simulink model "feedback_lin_RLS_Template_2023"  (R2023b)
settings: Solver=ode1  StartTime=0.0  StopTime=inf  FixedStep=0.002  RelTol=1e-3  EnableMultiTasking=on
PostLoadFcn:
  | qc_set_target_type(getConfigSet(bdroot, 'QUARC Default Target Configuration'));
values from neighbouring files (symbols this model uses):
  A_ob = A - L*C    [main_feedback_lin.m]
  B_ob = [ B - L*D, L]    [main_feedback_lin.m]
  C_ob = eye(n)    [main_feedback_lin.m]
  D_ob = zeros(n, q+p)    [main_feedback_lin.m]
  k_mag_mod = 3.4405e-05    [main_feedback_lin.m]
  Lc_mod = 0.3708    [main_feedback_lin.m]
  Rtot_mod = 7.7585    [main_feedback_lin.m]
undefined symbols (not defined in the file or in its folder): HIL, k_aero, k_mag, Kb, Lc, m, offset_corrente_volt, offset_posizione_volt, Rtot, x1_eq0, x2_eq0, y0
libraries: quarc_library x4, slpidlib x1
settings Model: SimulationMode=external  ExtModeTrigDuration=5000  Creator=CFulford  LastModifiedBy=lollo
settings SolverCC: AlgebraicLoopSolver=TrustRegion  PositivePriorityOrder=on
settings DataIOCC: LimitDataPoints=on  SaveFormat=Array  SignalLoggingSaveFormat=ModelDataLogs  ReturnWorkspaceOutputs=off
settings OptimizationCC: ExpressionDepthLimit=2147483647  InitFltsAndDblsToZero=on  LifeSpan=inf
settings DebuggingCC: SaveWithParameterizedLinksMsg=none  UnderspecifiedInitializationDetection=Classic  MergeDetectMultiDrivingBlocksExec=none  SolverPrmCheckMsg=warning  MultiTaskDSMMsg=warning  MultiTaskCondExecSysMsg=none  FcnCallInpInsideContextMsg=warning  UnconnectedInputMsg=warning  UnconnectedOutputMsg=warning  UnconnectedLineMsg=warning  StateNameClashWarn=warning  SFUnexpectedBacktrackingDiag=warning  SFNoUnconditionalDefaultTransitionDiag=warning  SFExecutionAtInitializationDiag=none  ArithmeticOperatorsInVariantConditions=warning
settings HardwareCC: ProdBitPerPointer=32  ProdBitPerSizeT=32  ProdBitPerPtrDiffT=32  ProdLargestAtomicFloat=None  ProdIntDivRoundTo=Undefined  ProdEndianess=Unspecified  ProdWordSize=32  ProdHWDeviceType=32-bit Generic
settings ModelReferenceCC: EnableRefExpFcnMdlSchedulingChecks=on  PropagateSignalLabelsOutOfModel=off
settings SFSimCC: SimUseLocalCustomCode=off  CustomCodeUndefinedFunction=UseInterfaceOnly
settings RTWCC: Description=QUARC Win64 Target  SystemTargetFile=quarc_win64.tlc  TemplateMakefile=quarc_default_tmf  RTWUseLocalCustomCode=off
settings CodeAppCC: StateflowObjectComments=on
settings STFCustomTargetCC: TargetPreCompLibLocation=C:\PROGRA~3\QUARC\lib\2019b\win64\release  TargetLangStandard=C89/C90 (ANSI)  ConcurrentExecutionCompliant=on  CombineOutputUpdateFcns=on  CPPClassGenCompliant=on  SystemTargetFile=quarc_win64.tlc
settings GRTTargetCC: TargetPreCompLibLocation=C:\PROGRA~3\QUARC\lib\2019b\win64\release  TargetLangStandard=C89/C90 (ANSI)  ParMdlRefBuildCompliant=off  CompOptLevelCompliant=off  MatFileLogging=off  UseToolchainInfoCompliant=off  ExtMode=on  ExtModeMexFile=quarc_comm
settings ConfigComp: CovMetricSettings=dw  CovSaveCumulativeToWorkspaceVar=on  CovSaveSingleToWorkspaceVar=on  CovExternalEMLEnable=off  CovSFcnEnable=off

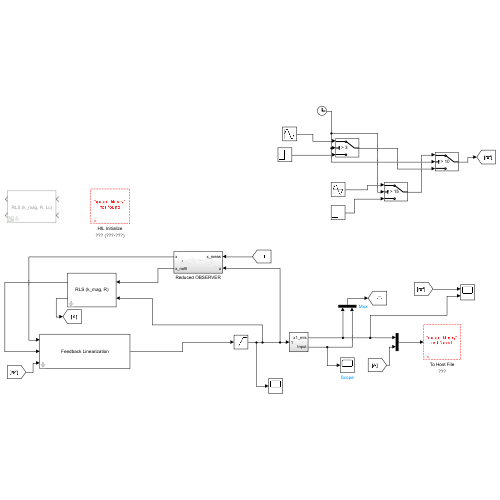
[thumbnail: Simulink's stored preview of the top-level diagram]
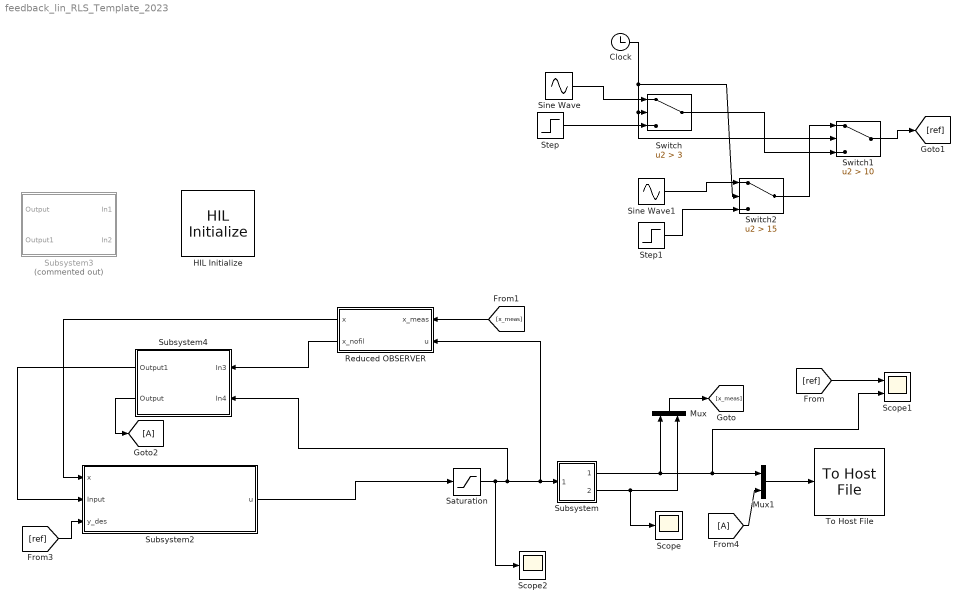
== system feedback_lin_RLS_Template_2023 ==
  Clock : Clock
  From4 : From
  Goto2 : Goto
  HIL Initialize : quarc_library/Data Acquisition/Generic/Configuration/HIL Initialize  Priority=-99  object_name=HIL-1  board_type=q2_usb  board_number=0  board_options=d0=digital;d1=digital;led=auto;update_rate=normal;decimation=1  exclusive=off  active=off  hardware_clocks=[0]  clock_modes=[]  initial_clock_frequencies=[]  set_clock_params_at_start=off  set_clock_params_at_switch_in=off  set_clock_frequencies_at_start=off  set_clock_frequencies_at_switch_in=off  analog_input_channels=[0:1]  analog_input_configurations=[]  analog_input_maximums=10  analog_input_minimums=-10  set_analog_input_params_at_start=on  set_analog_input_params_at_switch_in=off  analog_output_channels=[0:1]  analog_output_maximums=10  analog_output_minimums=-10  initial_analog_outputs=[0]  final_analog_outputs=[0]  watchdog_analog_outputs=0  set_analog_output_params_at_start=on  set_analog_output_params_at_switch_in=off  set_analog_outputs_at_start=on  set_analog_outputs_at_switch_in=off  set_analog_outputs_at_terminate=on  set_analog_outputs_at_switch_out=off  set_analog_outputs_on_watchdog=off  digital_input_channels=[]  digital_output_channels=[]  digital_output_configuration=[]  initial_digital_outputs=[1]  final_digital_outputs=[1]  watchdog_digital_outputs=[1]  set_digital_output_params_at_start=off  set_digital_output_params_at_switch_in=off  set_digital_outputs_at_start=on  set_digital_outputs_at_switch_in=off  set_digital_outputs_at_terminate=on  set_digital_outputs_at_switch_out=off  set_digital_outputs_on_watchdog=off  encoder_channels=[0:1]  quadrature=[4]  encoder_filter_frequency=[]  initial_encoder_counts=[0]  set_encoder_params_at_start=on  set_encoder_params_at_switch_in=off  set_encoder_counts_at_start=on  set_encoder_counts_at_switch_in=off  pwm_channels=[]  pwm_modes=[0]  pwm_frequency=1/0.020  pwm_configuration=[]  pwm_alignment=[]  pwm_polarity=[]  pwm_leading_deadband=[]  pwm_trailing_deadband=[]  initial_pwm_outputs=[0]  final_pwm_outputs=[0]  watchdog_pwm_outputs=[0]  set_pwm_params_at_start=on  set_pwm_params_at_switch_in=off  set_pwm_outputs_at_start=on  set_pwm_outputs_at_switch_in=off  set_pwm_outputs_at_terminate=on  set_pwm_outputs_at_switch_out=off  set_pwm_outputs_on_watchdog=off  other_output_channels=[]  initial_other_outputs=[]  final_other_outputs=[]  watchdog_other_outputs=[]  set_other_outputs_at_start=off  set_other_outputs_at_switch_in=off  set_other_outputs_at_terminate=off  set_other_outputs_at_switch_out=off  set_other_outputs_on_watchdog=off
  Mux : Mux  Inputs=2
  Mux1 : Mux  Inputs=2
  Reduced OBSERVER : Subsystem
  Saturation : Saturate  UpperLimit=23  LowerLimit=0
  Scope : Scope
  Scope1 : Scope  NumInputPorts=2
  Scope2 : Scope
  Sine Wave : Sin  Amplitude=0.0008  Bias=0.004  Frequency=10  SampleTime=0
  Sine Wave1 : Sin  Amplitude=0.0005  Bias=0.004  Frequency=10  SampleTime=0
  Step : Step  Time=2  After=0.004  SampleTime=0
  Step1 : Step  Time=2  After=0.003  SampleTime=0
  Subsystem : Subsystem
  Subsystem2 : Subsystem  mask{tau=0.003, p1=-100, p2=-60, p3=-70}
      mask DialogControl DescGroupVar Prompt: Feedback Linearization
      mask DialogControl DescTextVar Prompt: Tau corrisponde al tempo caratteristico del filtro per il calcolo delle derivate. k1, k2, k3 sono i poli della feedback linearization dei rispettivi stati
      mask Display: disp('Feedback Linearization')
  Subsystem3 : Subsystem  Commented=on
      mask Display: disp('RLS (k_mag, R, Lc)')
  Subsystem4 : Subsystem
      mask Display: disp('RLS (k_mag, R)')
  Switch : Switch  Criteria=u2 > Threshold  Threshold=3  SaturateOnIntegerOverflow=off  InputSameDT=off
  Switch1 : Switch  Criteria=u2 > Threshold  Threshold=10  SaturateOnIntegerOverflow=off  InputSameDT=off
  Switch2 : Switch  Criteria=u2 > Threshold  Threshold=15  SaturateOnIntegerOverflow=off  InputSameDT=off
  To Host File : quarc_library/Sinks/To Host/To Host File  file_name=data_%{date}_%{time}.mat  variable_name=data_%{date}_%{time}  decimation=1  sample_time=-1  file_format=MAT-file v.5  options=No header or footer  append=off  final_file_name=data_23-May-2025_13-05-44.mat  bitrate=2000000
  wires:
  Saturation/1 -> Scope2/1, Subsystem4/2(In4), Reduced OBSERVER/2(u), Subsystem/1(In1)
  Subsystem/2(Input) -> Mux/2, Scope/1
  Mux1/1 -> To Host File/1
  Subsystem2/1(u) -> Saturation/1
  [x_meas] -> Reduced OBSERVER/1(x_meas)
  Reduced OBSERVER/2(x_nofil) -> Subsystem4/1(In3)
  Reduced OBSERVER/1(x) -> Subsystem2/1(x)
  Subsystem4/1(Output1) -> Subsystem2/2(Input)
  Sine Wave/1 -> Switch/1
  Step/1 -> Switch/3
  [ref] -> Subsystem2/3(y_des)
  Subsystem4/2(Output) -> Goto2/1
  From4/1 -> Mux1/2
  Mux/1 -> [x_meas]
  Step1/1 -> Switch2/3
  Sine Wave1/1 -> Switch2/1
  Switch/1 -> Switch1/3
  Switch2/1 -> Switch1/1
  Clock/1 -> Switch1/2, Switch/2, Switch2/2
  Switch1/1 -> [ref]
  [ref] -> Scope1/1
  Subsystem/1(x1_mis) -> Scope1/2, Mux1/1, Mux/1

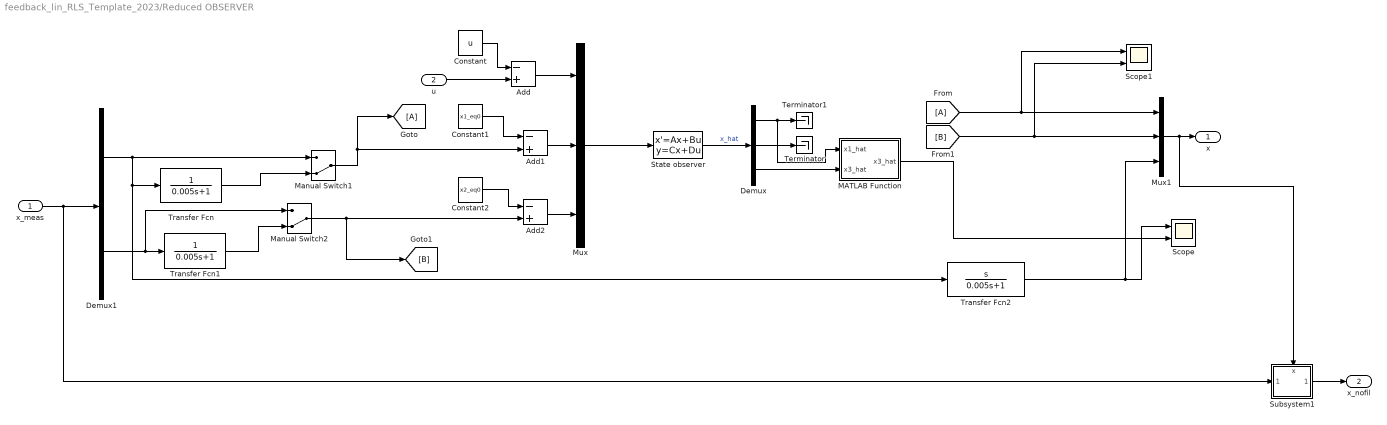
== system feedback_lin_RLS_Template_2023/Reduced OBSERVER ==
  x_meas : Inport
  u : Inport  Port=2
  Add : Sum  Inputs=-+
  Add1 : Sum  Inputs=-+
  Add2 : Sum  Inputs=-+
  Constant : Constant  Value=u
  Constant1 : Constant  Value=x1_eq0
  Constant2 : Constant  Value=x2_eq0
  Demux : Demux  Outputs=3
  Demux1 : Demux  Outputs=2
  From : From
  Goto : Goto
  MATLAB Function : MATLAB Function  TreatAsAtomicUnit=on
  Manual Switch1 : ManualSwitch  CurrentSetting=0
  Manual Switch2 : ManualSwitch  CurrentSetting=0
  Mux : Mux  Inputs=3
  Mux1 : Mux  Inputs=3
  Scope : Scope  NumInputPorts=2
  Scope1 : Scope  NumInputPorts=2
  State observer : StateSpace  A=A_ob  B=B_ob  C=C_ob  D=D_ob  InitialCondition=[0;0;0]
  Subsystem1 : Subsystem
      settings: PortSchema="{\"entries\":[{\"content\":{\"sides\":[{\"content\":{\"connectorIds\":[\"In1\"]},\"type\":\"ConnectorPlacement.EquallySpacedRectSide\",\"uuid\":\"f48180fa-4225-4978-addf-748f5b56b5ff\"},{\"content\":{\"connectorIds\":[\"Out1\"],\"side\":\"RIGHT\"},\"type\":\"ConnectorPlacement.EquallySpacedRectSide\",\"uuid\":\"29b082be-84d5-4b73-aaf8-582ec952e070\"},{\"content\":{\"connectorIds\":[\"In2\"],\"side\":\"TOP\"},\"type\":\"ConnectorPlacement.EquallySpacedRectSide\",\"uuid\":\"6e43ab95-1f09-4bed-ac58-60c8e8d5deec\"}]},\"type\":\"ConnectorPlacement.EquallySpacedConnector\",\"uuid\":\"d6520a9c-dc2f-4cc0-9c8c-cd26f1cfe6f6\"}],\"packageUris\":[\"http://schema.mathworks.com/mf0/Connector/R2020b\"],\"version\":\"1.0\"}"
  Terminator : Terminator
  Terminator1 : Terminator
  Transfer Fcn : TransferFcn  Denominator=[0.005 1]
  Transfer Fcn1 : TransferFcn  Denominator=[0.005 1]
  Transfer Fcn2 : TransferFcn  Numerator=[1 0]  Denominator=[0.005 1]
  x : Outport
  x_nofil : Outport  Port=2
  wires:
  u/1 -> Add/2
  Mux/1 -> State observer/1
  State observer/1 -> Demux/1  "x_hat"
  Demux/1 -> Terminator1/1, MATLAB Function/1(x1_hat)
  Constant/1 -> Add/1
  Constant1/1 -> Add1/1
  Constant2/1 -> Add2/1
  Add/1 -> Mux/1
  Add1/1 -> Mux/2
  Add2/1 -> Mux/3
  Demux/3 -> MATLAB Function/2("x3_hat ")
  Mux1/1 -> Subsystem1/2(x), x/1
  MATLAB Function/1(x3_hat) -> Scope/2
  Demux/2 -> Terminator/1
  x_meas/1 -> Subsystem1/1(x_meas), Demux1/1
  [B] -> Scope1/2, Mux1/2
  From/1 -> Scope1/1, Mux1/1
  Transfer Fcn/1 -> Manual Switch1/2
  Demux1/1 -> Transfer Fcn2/1, Transfer Fcn/1, Manual Switch1/1
  Manual Switch1/1 -> Add1/2, Goto/1
  Transfer Fcn1/1 -> Manual Switch2/2
  Demux1/2 -> Manual Switch2/1, Transfer Fcn1/1
  Manual Switch2/1 -> Add2/2, [B]
  Transfer Fcn2/1 -> Mux1/3, Scope/1
  Subsystem1/1(Out1) -> x_nofil/1

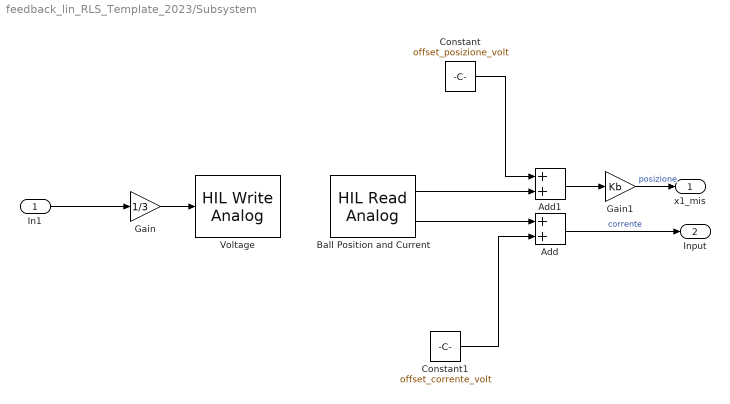
== system feedback_lin_RLS_Template_2023/Subsystem ==
  In1 : Inport
  Add : Sum
  Add1 : Sum
  Ball Position and Current : quarc_library/Data Acquisition/Generic/Immediate I//O/HIL Read Analog  object_name=HIL-1  channels=[0:1]  sample_time=qc_get_step_size  active=on  vector_output=off
  Constant : Constant  Value=offset_posizione_volt
  Constant1 : Constant  Value=offset_corrente_volt
  Gain : Gain  Gain=1/3
  Gain1 : Gain  Gain=Kb
  Voltage : quarc_library/Data Acquisition/Generic/Immediate I//O/HIL Write Analog  object_name=HIL-1  channels=0  sample_time=-1  active=off  vector_input=off
  x1_mis : Outport
  Input : Outport  Port=2
  wires:
  Ball Position and Current/1 -> Add1/2
  In1/1 -> Gain/1
  Ball Position and Current/2 -> Add/1
  Gain/1 -> Voltage/1
  Gain1/1 -> x1_mis/1  "posizione"
  Add1/1 -> Gain1/1
  Add/1 -> Input/1  "corrente"
  Constant1/1 -> Add/2
  Constant/1 -> Add1/1

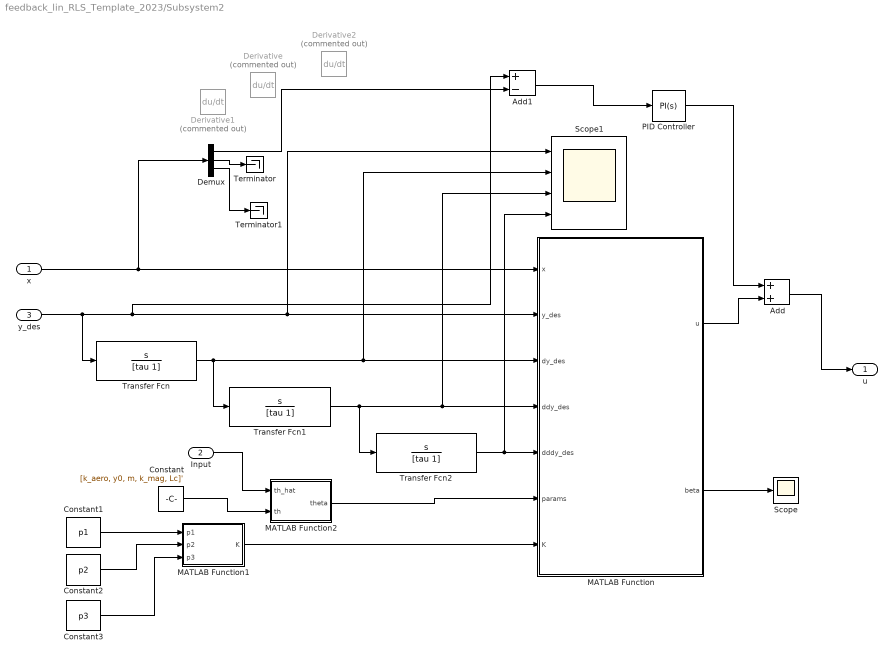
== system feedback_lin_RLS_Template_2023/Subsystem2 ==
  x : Inport
  Input : Inport  Port=2
  y_des : Inport  Port=3
  Add : Sum
  Add1 : Sum  Inputs=+-
  Constant : Constant  Value=[k_aero, y0, m, k_mag, Lc]'
  Constant1 : Constant  Value=p1
  Constant2 : Constant  Value=p2
  Constant3 : Constant  Value=p3
  Demux : Demux  Outputs=3
  Derivative : Derivative  Commented=on
  Derivative1 : Derivative  Commented=on
  Derivative2 : Derivative  Commented=on
  MATLAB Function : MATLAB Function  TreatAsAtomicUnit=on
  MATLAB Function1 : MATLAB Function  TreatAsAtomicUnit=on
  MATLAB Function2 : MATLAB Function  TreatAsAtomicUnit=on
  PID Controller : slpidlib/PID Controller  Controller=PI  Form=Parallel  TimeDomain=Continuous-time  UseExternalTs=off  SampleTime=-1  IntegratorMethod=Forward Euler  FilterMethod=Forward Euler  ControllerParametersSource=internal  P=1e2  I=3e3  UseKiTs=off  D=0  N=100  UseFilter=on  TunerSelectOption=Transfer Function Based (PID Tuner App)  InitialConditionSource=internal  InitialConditionForIntegrator=0  InitialConditionForFilter=0  DifferentiatorICPrevScaledInput=0  ExternalReset=none  TrackingMode=off  Kt=1  LimitOutput=off  SatLimitsSource=internal  UpperSaturationLimit=inf  LowerSaturationLimit=-inf  LinearizeAsGain=on  AntiWindupMode=none  Kb=1  LimitIntegrator=off  UpperIntegratorSaturationLimit=inf  LowerIntegratorSaturationLimit=-inf  POutMin=[]  POutMax=[]  IOutMin=[]  IOutMax=[]  DOutMin=[]  DOutMax=[]  NOutMin=[]  NOutMax=[]  SumOutMin=[]  SumOutMax=[]  SaturationOutMin=[]  SaturationOutMax=[]  PParamMin=[]  PParamMax=[]  IParamMin=[]  IParamMax=[]  DParamMin=[]  DParamMax=[]  NParamMin=[]  NParamMax=[]  KbParamMin=[]  KbParamMax=[]  KtParamMin=[]  KtParamMax=[]  KbOutMin=[]  KbOutMax=[]  KtOutMin=[]  KtOutMax=[]  IntegratorOutMin=[]  IntegratorOutMax=[]  FilterOutMin=[]  FilterOutMax=[]  SumI1OutMin=[]  SumI1OutMax=[]  SumI2OutMin=[]  SumI2OutMax=[]  SumI3OutMin=[]  SumI3OutMax=[]  SumI4OutMin=[]  SumI4OutMax=[]  SumDOutMin=[]  SumDOutMax=[]  DifferentiatorOutMin=[]  DifferentiatorOutMax=[]  FilterDiffOutCoefMin=[]  FilterDiffOutCoefMax=[]  ReciprocalOutMin=[]  ReciprocalOutMax=[]  SumDenOutMin=[]  SumDenOutMax=[]  SumNumOutMin=[]  SumNumOutMax=[]  DivideOutMin=[]  DivideOutMax=[]  UdiffTsProdOutMin=[]  UdiffTsProdOutMax=[]  NTsProdOutMin=[]  NTsProdOutMax=[]  UintegralTsProdOutMin=[]  UintegralTsProdOutMax=[]  UngainTsProdOutMin=[]  UngainTsProdOutMax=[]  ClampingZeroOutDataTypeStr=Inherit: Inherit via back propagation  ClampingZeroOutMin=[]  ClampingZeroOutMax=[]  FilterDenConstantOutDataTypeStr=Inherit: Inherit via back propagation  FilterDenConstantOutMin=[]  FilterDenConstantOutMax=[]  PCopyOutDataTypeStr=Inherit: Inherit via back propagation  PCopyOutMin=[]  PCopyOutMax=[]  NCopyOutDataTypeStr=Inherit: Inherit via back propagation  NCopyOutMin=[]  NCopyOutMax=[]  IntegratorContinuousStateAttributes=''  IntegratorStateMustResolveToSignalObject=off  IntegratorRTWStateStorageClass=Auto  FilterContinuousStateAttributes=''  FilterStateMustResolveToSignalObject=off  FilterRTWStateStorageClass=Auto  ParallelPVariant=InternalParameters  IdealPVariant=Disabled  IVariant=InternalParameters  DVariant=Disabled  IntegratorVariant=Continuous  SatVariant=Disabled  AWVariant=Passthrough  PCopyVariant=Disabled  TRVariant=Disabled  FdbkBlocksVariant=Forward  IdealPFdbkVariant=Disabled  SatFdbkVariant=Disabled  DerivativeFilterVariant=Disabled  NVariant=Disabled  NCopyVariant=Disabled_SignalSpec  FilterICVariant=Disabled  IntegratorICVariant=InternalICs  ExternalResetVariant=Disabled  TRSumVariant=Passthrough  SumFdbkVariant=Disabled  SumVariant=Sum_PI  TsampFilterVariant=InternalTs  TsampNgainVariant=Passthrough  TsampIntegralVariant=Disabled_SignalSpec  ExternalSaturationOutDataTypeStr=Inherit: Same as second input
  Scope : Scope
  Scope1 : Scope  NumInputPorts=4
  Terminator : Terminator
  Terminator1 : Terminator
  Transfer Fcn : TransferFcn  Numerator=[1 0]  Denominator=[tau 1]
  Transfer Fcn1 : TransferFcn  Numerator=[1 0]  Denominator=[tau 1]
  Transfer Fcn2 : TransferFcn  Numerator=[1 0]  Denominator=[tau 1]
  u : Outport
  wires:
  y_des/1 -> Transfer Fcn/1, Add1/1, MATLAB Function/2(y_des), Scope1/1
  x/1 -> Demux/1, MATLAB Function/1(x)
  MATLAB Function/1(u) -> Add/2
  Transfer Fcn/1 -> MATLAB Function/3(dy_des), Scope1/2, Transfer Fcn1/1
  MATLAB Function2/1(theta) -> MATLAB Function/6(params)
  Transfer Fcn1/1 -> Transfer Fcn2/1, Scope1/3, MATLAB Function/4(ddy_des)
  MATLAB Function/2(beta) -> Scope/1
  Transfer Fcn2/1 -> Scope1/4, MATLAB Function/5(dddy_des)
  MATLAB Function1/1(K) -> MATLAB Function/7(K)
  Constant3/1 -> MATLAB Function1/3(p3)
  Constant2/1 -> MATLAB Function1/2(p2)
  Constant1/1 -> MATLAB Function1/1(p1)
  Input/1 -> MATLAB Function2/1(th_hat)
  Constant/1 -> MATLAB Function2/2(th)
  Add/1 -> u/1
  PID Controller/1 -> Add/1
  Demux/1 -> Add1/2
  Demux/2 -> Terminator/1
  Demux/3 -> Terminator1/1
  Add1/1 -> PID Controller/1

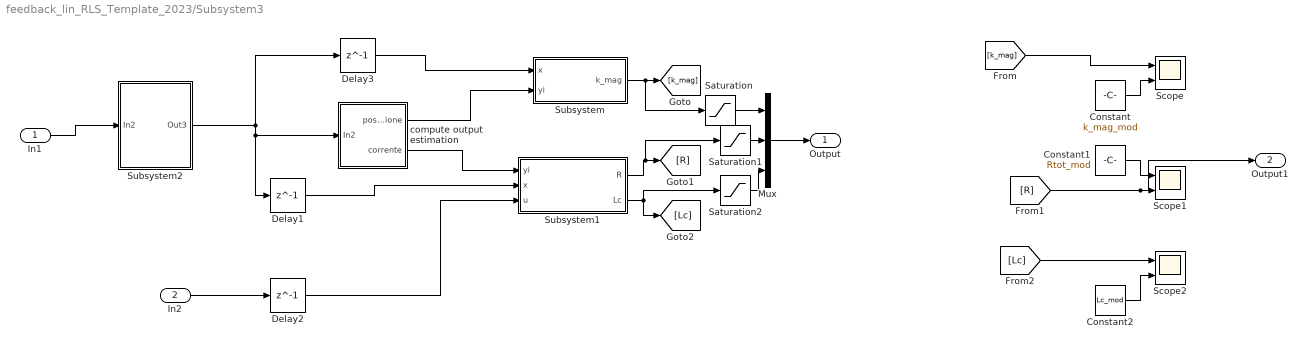
== system feedback_lin_RLS_Template_2023/Subsystem3 ==
  In1 : Inport
  In2 : Inport  Port=2
  Constant : Constant  Value=k_mag_mod
  Constant1 : Constant  Value=Rtot_mod
  Constant2 : Constant  Value=Lc_mod
  Delay1 : Delay  DelayLength=1  InitialCondition=0
  Delay2 : Delay  DelayLength=1  InitialCondition=0
  Delay3 : Delay  DelayLength=1  InitialCondition=[0, 0, 0]'
  Mux : Mux  Inputs=3
  Saturation : Saturate  UpperLimit=1e-4  LowerLimit=1e-6
  Saturation1 : Saturate  UpperLimit=13  LowerLimit=0
  Saturation2 : Saturate  UpperLimit=2  LowerLimit=0
  Scope : Scope  NumInputPorts=2
  Scope1 : Scope  NumInputPorts=2
  Scope2 : Scope  NumInputPorts=2
  Subsystem : Subsystem  mask{th0=k_mag, S0=eye(1)/100, mu=0.98}
      mask prompts: th0 "Theta init"; mu "Forgetting factor"
      mask Display: disp('RLS (k_mag)')
  Subsystem1 : Subsystem  mask{th0=[Rtot; Lc], S0=eye(2)/10, mu=0.99}
      mask prompts: th0 "Theta init"; mu "Forgetting Factor"
      mask Display: disp('RLS (R, Lc)')
  Subsystem2 : Subsystem
  compute output estimation : Subsystem
  Output : Outport
  Output1 : Outport  Port=2
  wires:
  In2/1 -> Delay2/1
  Delay2/1 -> Subsystem1/3(u)
  Delay3/1 -> Subsystem/1(x)
  compute output estimation/1(posizione) -> Subsystem/2(yi)
  compute output estimation/2(corrente) -> Subsystem1/1(yi)
  Delay1/1 -> Subsystem1/2(x)
  Constant/1 -> Scope/2
  Constant1/1 -> Scope1/1
  Constant2/1 -> Scope2/2
  Subsystem/1(k_mag) -> Saturation/1, [k_mag]
  Subsystem1/1(R) -> Saturation1/1, [R]
  Subsystem1/2(Lc) -> [Lc], Saturation2/1
  [k_mag] -> Scope/1
  [R] -> Output1/1, Scope1/2
  [Lc] -> Scope2/1
  Mux/1 -> Output/1
  Subsystem2/1(Out3) -> Delay1/1, compute output estimation/1(In2), Delay3/1
  In1/1 -> Subsystem2/1(In2)
  Saturation/1 -> Mux/1
  Saturation1/1 -> Mux/2
  Saturation2/1 -> Mux/3

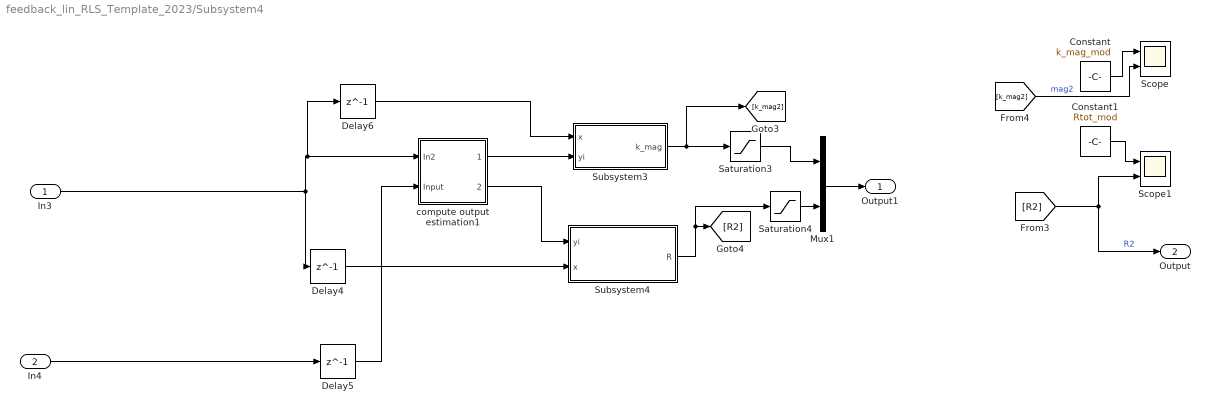
== system feedback_lin_RLS_Template_2023/Subsystem4 ==
  In3 : Inport
  In4 : Inport  Port=2
  Constant : Constant  Value=k_mag_mod
  Constant1 : Constant  Value=Rtot_mod
  Delay4 : Delay  DelayLength=1  InitialCondition=0
  Delay5 : Delay  DelayLength=1  InitialCondition=0
  Delay6 : Delay  DelayLength=1  InitialCondition=[0, 0, 0]'
  Mux1 : Mux  Inputs=2
  Saturation3 : Saturate  UpperLimit=1e-4  LowerLimit=1e-6
  Saturation4 : Saturate  UpperLimit=20  LowerLimit=0
  Scope : Scope  NumInputPorts=2
  Scope1 : Scope  NumInputPorts=2
  Subsystem3 : Subsystem  mask{th0=k_mag, S0=eye(1)/100, mu=0.98}
      mask prompts: th0 "Theta init"; mu "Forgetting factor"
      mask Display: disp('RLS (k_mag)')
  Subsystem4 : Subsystem  mask{th0=Rtot, S0=eye(1)/10, mu=0.99}
      mask prompts: th0 "Theta init"; mu "Forgetting Factor"
      mask Display: disp('RLS (R, Lc)')
  compute output estimation1 : Subsystem
  Output1 : Outport
  Output : Outport  Port=2
  wires:
  Constant/1 -> Scope/1
  Constant1/1 -> Scope1/1
  In3/1 -> Delay4/1, Delay6/1, compute output estimation1/1(In2)
  Saturation4/1 -> Mux1/2
  Subsystem4/1(R) -> Saturation4/1, [R2]
  Delay4/1 -> Subsystem4/2(x)
  Mux1/1 -> Output1/1
  compute output estimation1/2(corrente) -> Subsystem4/1(yi)
  In4/1 -> Delay5/1
  Delay5/1 -> compute output estimation1/2(Input)
  compute output estimation1/1(posizione) -> Subsystem3/2(yi)
  Subsystem3/1(k_mag) -> [k_mag2], Saturation3/1
  Saturation3/1 -> Mux1/1
  Delay6/1 -> Subsystem3/1(x)
  [R2] -> Scope1/2, Output/1  "R2"
  [k_mag2] -> Scope/2  "mag2"

== system feedback_lin_RLS_Template_2023/Reduced OBSERVER/Subsystem1 ==
  x_meas : Inport
  x : Inport  Port=2
  Demux : Demux  Outputs=2
  Demux1 : Demux  Outputs=3
  Mux : Mux  Inputs=3
  Terminator1 : Terminator
  Terminator2 : Terminator
  Out1 : Outport
  wires:
  x/1 -> Demux1/1
  x_meas/1 -> Demux/1
  Demux1/1 -> Terminator1/1
  Demux1/2 -> Terminator2/1
  Mux/1 -> Out1/1
  Demux/1 -> Mux/1
  Demux/2 -> Mux/2
  Demux1/3 -> Mux/3

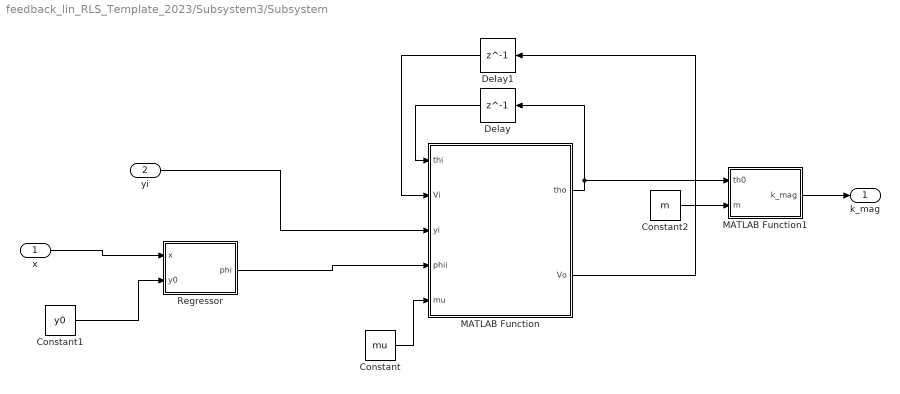
== system feedback_lin_RLS_Template_2023/Subsystem3/Subsystem ==
  x : Inport
  yi : Inport  Port=2
  Constant : Constant  Value=mu
  Constant1 : Constant  Value=y0
  Constant2 : Constant  Value=m
  Delay : Delay  DelayLength=1  InitialCondition=th0*0.002^2/m
  Delay1 : Delay  DelayLength=1  InitialCondition=inv(S0)
  MATLAB Function : MATLAB Function  TreatAsAtomicUnit=on
  MATLAB Function1 : MATLAB Function  TreatAsAtomicUnit=on
  Regressor : MATLAB Function  TreatAsAtomicUnit=on
  k_mag : Outport
  wires:
  yi/1 -> MATLAB Function/3(yi)
  Constant/1 -> MATLAB Function/5(mu)
  Delay/1 -> MATLAB Function/1(thi)
  Delay1/1 -> MATLAB Function/2(Vi)
  MATLAB Function/1(tho) -> MATLAB Function1/1(th0), Delay/1
  Regressor/1(phi) -> MATLAB Function/4(phii)
  MATLAB Function/2(Vo) -> Delay1/1
  x/1 -> Regressor/1(x)
  Constant1/1 -> Regressor/2(y0)
  MATLAB Function1/1(k_mag) -> k_mag/1
  Constant2/1 -> MATLAB Function1/2(m)

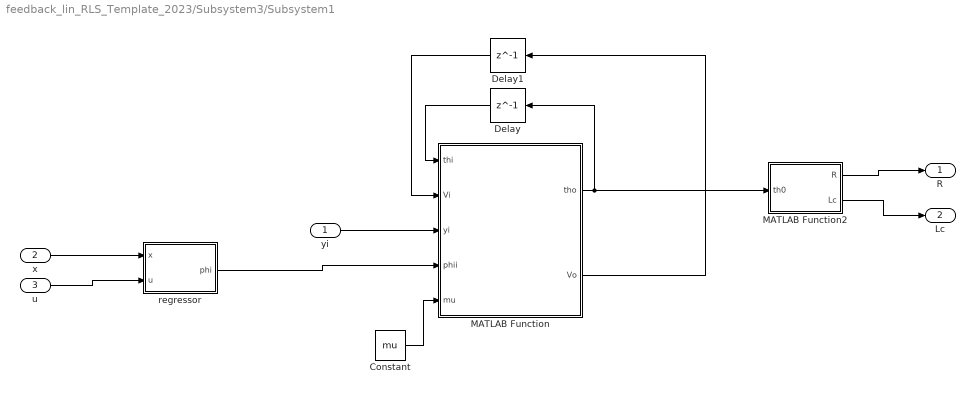
== system feedback_lin_RLS_Template_2023/Subsystem3/Subsystem1 ==
  yi : Inport
  x : Inport  Port=2
  u : Inport  Port=3
  Constant : Constant  Value=mu
  Delay : Delay  DelayLength=1  InitialCondition=[th0(1)*0.002/th0(2); 0.002/th0(2)]
  Delay1 : Delay  DelayLength=1  InitialCondition=inv(S0)
  MATLAB Function : MATLAB Function  TreatAsAtomicUnit=on
  MATLAB Function2 : MATLAB Function  TreatAsAtomicUnit=on
  regressor : MATLAB Function  TreatAsAtomicUnit=on
  R : Outport
  Lc : Outport  Port=2
  wires:
  yi/1 -> MATLAB Function/3(yi)
  Constant/1 -> MATLAB Function/5(mu)
  Delay/1 -> MATLAB Function/1(thi)
  Delay1/1 -> MATLAB Function/2(Vi)
  MATLAB Function/1(tho) -> MATLAB Function2/1(th0), Delay/1
  regressor/1(phi) -> MATLAB Function/4(phii)
  MATLAB Function/2(Vo) -> Delay1/1
  x/1 -> regressor/1(x)
  u/1 -> regressor/2(u)
  MATLAB Function2/1(R) -> R/1
  MATLAB Function2/2(Lc) -> Lc/1

== system feedback_lin_RLS_Template_2023/Subsystem3/Subsystem2 ==
  In2 : Inport
  Demux : Demux  Outputs=3
  Mux1 : Mux  Inputs=3
  Out3 : Outport
  wires:
  Mux1/1 -> Out3/1
  In2/1 -> Demux/1
  Demux/3 -> Mux1/3
  Demux/2 -> Mux1/2
  Demux/1 -> Mux1/1

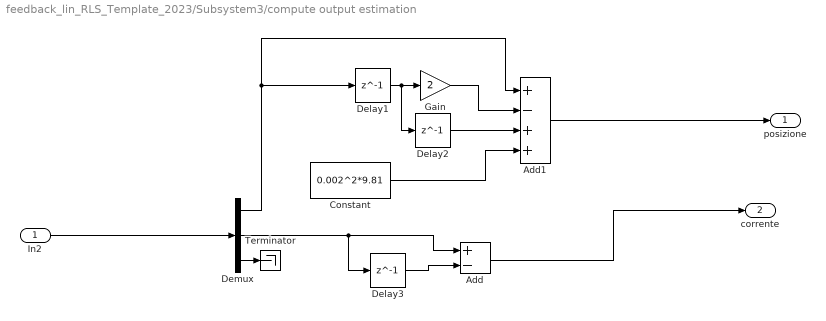
== system feedback_lin_RLS_Template_2023/Subsystem3/compute output estimation ==
  In2 : Inport
  Add : Sum  Inputs=+-
  Add1 : Sum  Inputs=+-++
  Constant : Constant  Value=0.002^2*9.81
  Delay1 : Delay  DelayLength=1
  Delay2 : Delay  DelayLength=1
  Delay3 : Delay  DelayLength=1
  Demux : Demux  Outputs=3
  Gain : Gain  Gain=2
  Terminator : Terminator
  posizione : Outport
  corrente : Outport  Port=2
  wires:
  In2/1 -> Demux/1
  Demux/3 -> Terminator/1
  Demux/2 -> Delay3/1, Add/1
  Delay3/1 -> Add/2
  Add/1 -> corrente/1
  Demux/1 -> Delay1/1, Add1/1
  Delay1/1 -> Delay2/1, Gain/1
  Gain/1 -> Add1/2
  Delay2/1 -> Add1/3
  Constant/1 -> Add1/4
  Add1/1 -> posizione/1

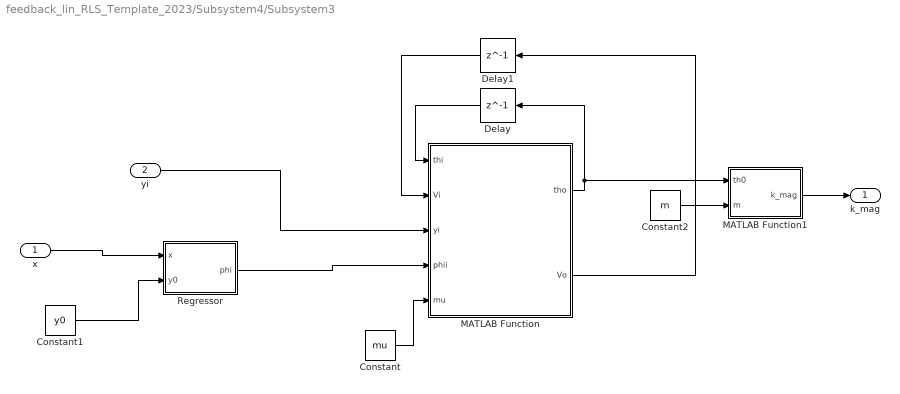
== system feedback_lin_RLS_Template_2023/Subsystem4/Subsystem3 ==
  x : Inport
  yi : Inport  Port=2
  Constant : Constant  Value=mu
  Constant1 : Constant  Value=y0
  Constant2 : Constant  Value=m
  Delay : Delay  DelayLength=1  InitialCondition=th0*0.002^2/m
  Delay1 : Delay  DelayLength=1  InitialCondition=inv(S0)
  MATLAB Function : MATLAB Function  TreatAsAtomicUnit=on
  MATLAB Function1 : MATLAB Function  TreatAsAtomicUnit=on
  Regressor : MATLAB Function  TreatAsAtomicUnit=on
  k_mag : Outport
  wires:
  yi/1 -> MATLAB Function/3(yi)
  Constant/1 -> MATLAB Function/5(mu)
  Delay/1 -> MATLAB Function/1(thi)
  Delay1/1 -> MATLAB Function/2(Vi)
  MATLAB Function/1(tho) -> MATLAB Function1/1(th0), Delay/1
  Regressor/1(phi) -> MATLAB Function/4(phii)
  MATLAB Function/2(Vo) -> Delay1/1
  x/1 -> Regressor/1(x)
  Constant1/1 -> Regressor/2(y0)
  MATLAB Function1/1(k_mag) -> k_mag/1
  Constant2/1 -> MATLAB Function1/2(m)

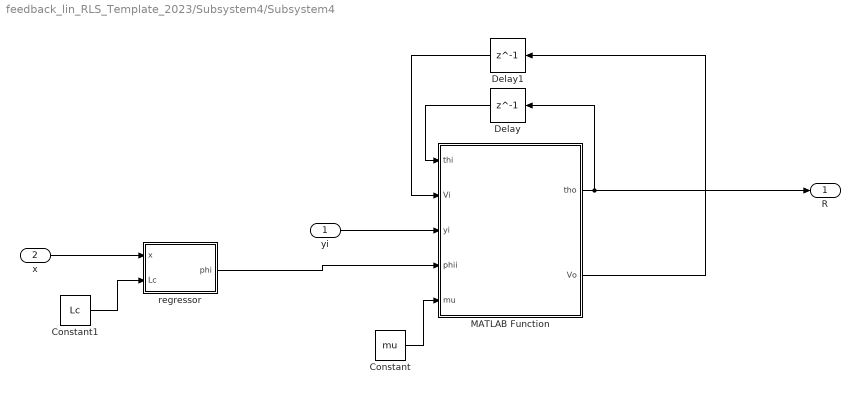
== system feedback_lin_RLS_Template_2023/Subsystem4/Subsystem4 ==
  yi : Inport
  x : Inport  Port=2
  Constant : Constant  Value=mu
  Constant1 : Constant  Value=Lc
  Delay : Delay  DelayLength=1  InitialCondition=th0
  Delay1 : Delay  DelayLength=1  InitialCondition=inv(S0)
  MATLAB Function : MATLAB Function  TreatAsAtomicUnit=on
  regressor : MATLAB Function  TreatAsAtomicUnit=on
  R : Outport
  wires:
  yi/1 -> MATLAB Function/3(yi)
  Constant/1 -> MATLAB Function/5(mu)
  Delay/1 -> MATLAB Function/1(thi)
  Delay1/1 -> MATLAB Function/2(Vi)
  regressor/1(phi) -> MATLAB Function/4(phii)
  MATLAB Function/2(Vo) -> Delay1/1
  x/1 -> regressor/1(x)
  MATLAB Function/1(tho) -> R/1, Delay/1
  Constant1/1 -> regressor/2(Lc)

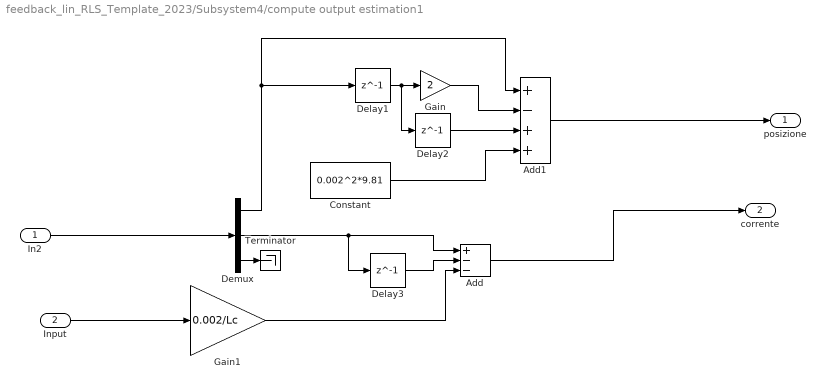
== system feedback_lin_RLS_Template_2023/Subsystem4/compute output estimation1 ==
  In2 : Inport
  Input : Inport  Port=2
  Add : Sum  Inputs=+--
  Add1 : Sum  Inputs=+-++
  Constant : Constant  Value=0.002^2*9.81
  Delay1 : Delay  DelayLength=1
  Delay2 : Delay  DelayLength=1
  Delay3 : Delay  DelayLength=1
  Demux : Demux  Outputs=3
  Gain : Gain  Gain=2
  Gain1 : Gain  Gain=0.002/Lc
  Terminator : Terminator
  posizione : Outport
  corrente : Outport  Port=2
  wires:
  In2/1 -> Demux/1
  Demux/3 -> Terminator/1
  Demux/2 -> Delay3/1, Add/1
  Delay3/1 -> Add/2
  Add/1 -> corrente/1
  Demux/1 -> Delay1/1, Add1/1
  Delay1/1 -> Delay2/1, Gain/1
  Gain/1 -> Add1/2
  Delay2/1 -> Add1/3
  Constant/1 -> Add1/4
  Add1/1 -> posizione/1
  Gain1/1 -> Add/3
  Input/1 -> Gain1/1

== matlab function feedback_lin_RLS_Template_2023/Subsystem2/MATLAB Function2 ==
  data: th_hat input; theta output; th input
function theta = fcn(th_hat, th)

%     k_mag = th_hat(1);
    Rtot = th_hat(2);
%     Lc = th_hat(3);
    k_aero = th(1);
    y0 = th(2);
    m = th(3);
    k_mag = th(4);
    Lc = th(5);

    theta = [k_aero, k_mag, m, y0, Rtot, Lc]';


end

== matlab function feedback_lin_RLS_Template_2023/Subsystem4/Subsystem3/MATLAB Function ==
  data: thi input; tho output; Vi input; yi input; phii input; Vo output; mu input
function [tho,Vo] = updaterule(thi,Vi,yi,phii,mu)

Vo = Vi/mu - (Vi*phii*phii'*Vi)/(mu+phii'*Vi*phii)/mu;
tho = thi + Vo*phii*(yi-phii'*thi);

== matlab function feedback_lin_RLS_Template_2023/Subsystem4/Subsystem3/MATLAB Function1 ==
  data: th0 input; k_mag output; m input
function k_mag = fcn(th0, m)

    k_mag = th0*m/0.002^2;



end

== matlab function feedback_lin_RLS_Template_2023/Subsystem4/Subsystem3/Regressor ==
  data: x input; phi output; y0 input
function phi = fcn(x, y0)
    
    phi = (x(2)/(y0 - x(1)))^2;
    
end

== matlab function feedback_lin_RLS_Template_2023/Subsystem4/Subsystem4/MATLAB Function ==
  data: thi input; tho output; Vi input; yi input; phii input; Vo output; mu input
function [tho,Vo] = updaterule(thi,Vi,yi,phii,mu)

Vo = Vi/mu - (Vi*phii*phii'*Vi)/(mu+phii'*Vi*phii)/mu;
tho = thi + Vo*phii*(yi-phii'*thi);

== matlab function feedback_lin_RLS_Template_2023/Reduced OBSERVER/MATLAB Function ==
  data: x1_hat input; x3_hat output; x3_hat input
function x3_hat = fcn(x1_hat, x3_hat)

    if x1_hat<=0 && x3_hat<=0
        x3_hat=0;
    end
end

== matlab function feedback_lin_RLS_Template_2023/Subsystem4/Subsystem4/regressor ==
  data: x input; Lc input; phi output
function phi = fcn(x, Lc)

    phi = -x(2)*0.002/Lc;

end

== matlab function feedback_lin_RLS_Template_2023/Subsystem3/Subsystem/MATLAB Function ==
  data: thi input; tho output; Vi input; yi input; phii input; Vo output; mu input
function [tho,Vo] = updaterule(thi,Vi,yi,phii,mu)

Vo = Vi/mu - (Vi*phii*phii'*Vi)/(mu+phii'*Vi*phii)/mu;
tho = thi + Vo*phii*(yi-phii'*thi);

== matlab function feedback_lin_RLS_Template_2023/Subsystem3/Subsystem/Regressor ==
  data: x input; phi output; y0 input
function phi = fcn(x, y0)
    
    phi = (x(2)/(y0 - x(1)))^2;
    
end

== matlab function feedback_lin_RLS_Template_2023/Subsystem3/Subsystem1/MATLAB Function ==
  data: thi input; tho output; Vi input; yi input; phii input; Vo output; mu input
function [tho,Vo] = updaterule(thi,Vi,yi,phii,mu)

Vo = Vi/mu - (Vi*phii*phii'*Vi)/(mu+phii'*Vi*phii)/mu;
tho = thi + Vo*phii*(yi-phii'*thi);

== matlab function feedback_lin_RLS_Template_2023/Subsystem3/Subsystem1/regressor ==
  data: x input; u input; phi output
function phi = fcn(x, u)

    phi = [-x(2); u];

end

== matlab function feedback_lin_RLS_Template_2023/Subsystem3/Subsystem1/MATLAB Function2 ==
  data: th0 input; R output; Lc output
function [R, Lc] = fcn(th0)

    R = th0(1)/th0(2);
    Lc = 0.002/th0(2);



end

== matlab function feedback_lin_RLS_Template_2023/Subsystem3/Subsystem/MATLAB Function1 ==
  data: th0 input; k_mag output; m input
function k_mag = fcn(th0, m)

    k_mag = th0*m/0.002^2;



end

== matlab function feedback_lin_RLS_Template_2023/Subsystem2/MATLAB Function ==
  data: x input; u output; y_des input; dy_des input; ddy_des input; dddy_des input; params input; K input; beta output

function [u, beta] = feedback_linearization_control(x, y_des, dy_des, ddy_des, dddy_des, params, K)
    % Estrai parametri
    k_aero = params(1);
    k_mag  = params(2);
    m      = params(3);
    y0     = params(4);
    Rtot   = params(5);
    Lc     = params(6);
    g      = 9.81;

    % Stati
    x1 = x(1); % posizione
    x2 = x(2); % corrente
    x3 = x(3); % velocità

    % Derivate
    denom = (y0 - x1);
%     if denom <= 0
%         warning('Denominatore nullo o negativo: instabilità elettromagnetica');
%     end

    % Accelerazione reale
    xdot3 = (k_aero/m)*x3 + (k_mag/m)*(x2 / denom)^2 - g;

    % Derivate parziali
    dBdx1 = (2 * k_mag * x2^2) / (m * denom^3);
    dBdx2 = (2 * k_mag * x2)   / (m * denom^2);
    dBdx3 = (k_aero/m);

    % Corrente senza ingresso (per calcolo alpha)
    dx2_nou = -(Rtot/Lc)*x2;

    % Parte non lineare (α) e lineare (β)
    alpha = dBdx1 * x3 + dBdx2 * dx2_nou + dBdx3 * xdot3;
    beta  = dBdx2 * (1/Lc);

%     if abs(beta) < 1e-6
%         warning('Beta troppo piccolo: possibile instabilità numerica');
%         u = 5;
%         return;
%     end

    % Errore e controllore
    e   = x1 - y_des;
    de  = x3 - dy_des;
    ae  = xdot3 - ddy_des;

    

    % Guadagni
    k1 = K(1);
    k2 = K(2);
    k3 = K(3);
    

    % Ingresso virtuale
    % v = p(1, 1)*dddy_des + p(1, 2)*e + p(1, 3)*de + p(1, 4)*ae;
    v = dddy_des - k1*e - k2*de - k3*ae;
    % v = -k1*x1 - k2*x2 - k3*x3;

    % Controllo reale
    u = (v - alpha) / beta;
end

== matlab function feedback_lin_RLS_Template_2023/Subsystem2/MATLAB Function1 ==
  data: p1 input; K output; p2 input; p3 input
function K = fcn(p1, p2, p3)

    desired_roots = [p1, p2, p3];
    coeff = poly(desired_roots);     % s^3 + a2*s^2 + a1*s + a0
    K = fliplr(coeff(2:end));
